simulink subsystem "stack_model_subsystem"  (R2023a)
settings: Solver=VariableStepAuto  StartTime=0.0  StopTime=10.0  RelTol=1e-3
undefined symbols (not defined in the file): constants, coolant_initial_temperature, dewpoint_temperature_degC, env_p, h2_molar_concentration, hydrogen, inlet_flow_lpmin, inlet_pressure_barg, inlet_temperature_degC, oxygen, stack, stack_num_cells, stoichiometry
libraries: fl_lib x28, nesl_utility x26
(part 1 of 2)
settings Model: Creator=stefan.notter  LastModifiedBy=adrian.taveras
settings OptimizationCC: ReuseModelBlockBuffer=off

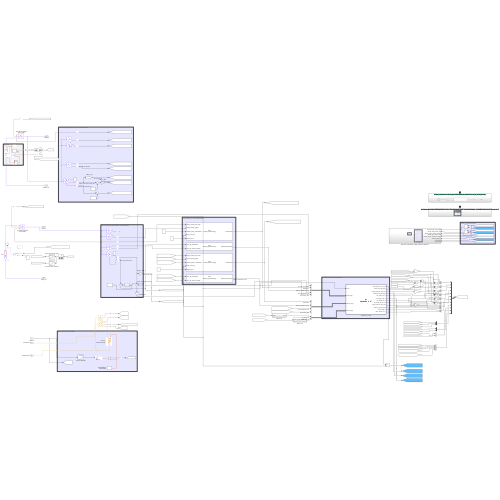
[thumbnail: Simulink's stored preview of the top-level diagram]
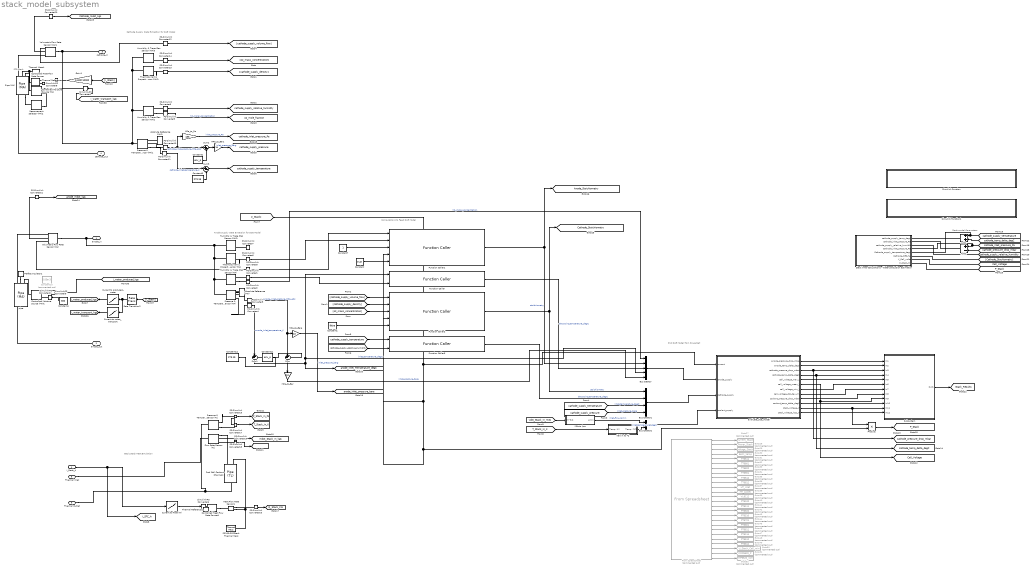
== system stack_model_subsystem ==
  note: Basic Stack Heat Emulation
  note: Computations to Feed DoE Model
  note: Anode Supply Data Extraction for DoE Model
  note: P10 DoE Model from PowerCell
  note: Cathode Supply Data Extraction for DoE Model
  note: FCS-Stack
  note: Stack-model-Parameters
  I_Stack_A : Inport
  Absolute Reference (MA) : fl_lib/Moist Air/Elements/Absolute Reference (MA)
  Absolute Reference (MA)1 : fl_lib/Moist Air/Elements/Absolute Reference (MA)
  Add1 : Sum
  Add2 : Sum  Inputs=+-
  Bus Creator : BusCreator  Inputs=h2_molar_concentration,stoichiometry,dewpoint_temperature_degC,inlet_temperature_degC,inlet_pressure_barg  OutDataTypeStr=Bus: anode_supply
  Bus Creator1 : BusCreator  Inputs=stoichiometry,dewpoint_temperature_degC,inlet_temperature_degC,inlet_pressure_barg  OutDataTypeStr=Bus: cathode_supply
  Bus Creator2 : BusCreator  Inputs=inlet_flow_lpmin,inlet_temperature_degC  OutDataTypeStr=Bus: coolant_supply
  Constant : Constant  Value=true  OutDataTypeStr=boolean
  Constant1 : Constant  Value=false  OutDataTypeStr=boolean
  Constant10 : Constant  Commented=on  Value=0.05e-3
  Constant11 : Constant  Value=env_p
  Constant12 : Constant  Value=273.15
  Constant2 : Constant  Value=env_p
  Constant3 : Constant  Value=273.15
  Constant4 : Constant  Value=300
  Constant7 : Constant
  Controlled Heat Flow Rate Source : fl_lib/Thermal/Thermal Sources/Controlled Heat Flow Rate Source
  Controlled Heat Flow Rate Source1 : fl_lib/Thermal/Thermal Sources/Controlled Heat Flow Rate Source
  Controlled Moisture Source (MA) : fl_lib/Moist Air/Sources/Moisture & Trace Gas Sources/Controlled Moisture Source (MA)  moisture_source_spec=foundation.enum.moisture_source_spec.vapor  Phi_S_specify=off  Phi_S_priority=None  Phi_S=0 kW  Phi_S_nominal_specify=off  Phi_S_nominal_unit=kW  Phi_S_nominal_value=1  mdot_w_S_specify=off  mdot_w_S_priority=None  mdot_w_S=0 kg/s  mdot_w_S_nominal_specify=off  mdot_w_S_nominal_unit=kg/s  mdot_w_S_nominal_value=1
      settings: InternalSimscapePortConfiguration="{\"Bottom\":[],\"Left\":[{\"id\":\"S\",\"label\":\"S\",\"type\":\"foundation.moist_air.moist_air_source\"}],\"Right\":[{\"id\":\"M\",\"label\":\"M\",\"type\":\"input\"},{\"id\":\"T\",\"label\":\"T\",\"type\":\"input\"}],\"Top\":[]}"
  Controlled Moisture Source (MA)1 : fl_lib/Moist Air/Sources/Moisture & Trace Gas Sources/Controlled Moisture Source (MA)  moisture_source_spec=foundation.enum.moisture_source_spec.vapor  Phi_S_specify=off  Phi_S_priority=None  Phi_S=0 kW  Phi_S_nominal_specify=off  Phi_S_nominal_unit=kW  Phi_S_nominal_value=1  mdot_w_S_specify=off  mdot_w_S_priority=None  mdot_w_S=0 kg/s  mdot_w_S_nominal_specify=off  mdot_w_S_nominal_unit=kg/s  mdot_w_S_nominal_value=1
      settings: InternalSimscapePortConfiguration="{\"Bottom\":[],\"Left\":[{\"id\":\"S\",\"label\":\"S\",\"type\":\"foundation.moist_air.moist_air_source\"}],\"Right\":[{\"id\":\"M\",\"label\":\"M\",\"type\":\"input\"},{\"id\":\"T\",\"label\":\"T\",\"type\":\"input\"}],\"Top\":[]}"
  Current to Heat (W) : Lookup_n-D  NumberOfTableDimensions=1  BreakpointsForDimension1=[0:50:400]  Table=[0, 9932, 21438, 33442,47123, 59491, 77033, 93585, 112042]  InternalRulePriority=Speed  RndMeth=Simplest
  Current to produced_water : Lookup_n-D  NumberOfTableDimensions=1  BreakpointsForDimension1=[0;100;200;400;600]  Table=[0;6.491e-6;1.132e-5;1.762e-5;2.762e-5]  InternalRulePriority=Speed  RndMeth=Simplest
  Current to water_transport : Lookup_n-D  NumberOfTableDimensions=1  BreakpointsForDimension1=[0;100;200;400;600]  Table=[0;4.247e-3;8.494e-3;1.697e-2;2.548e-2]  InternalRulePriority=Speed  RndMeth=Simplest
  Flow Rate Sensor (TL) : fl_lib/Thermal Liquid/Sensors/Flow Rate Sensor (TL)  mass_flow_measure=true  volumetric_flow_measure=true  energy_flow_measure=false
      settings: InternalSimscapePortConfiguration="{\"Bottom\":[],\"Left\":[{\"id\":\"A\",\"label\":\"A\",\"type\":\"foundation.thermal_liquid.thermal_liquid\"}],\"Right\":[{\"id\":\"B\",\"label\":\"B\",\"type\":\"foundation.thermal_liquid.thermal_liquid\"},{\"id\":\"M\",\"label\":\"M\",\"type\":\"output\"},{\"id\":\"V\",\"label\":\"V\",\"type\":\"output\"}],\"Top\":[]}"
  From Spreadsheet : FromSpreadsheet  Commented=on  FileName=20231018_14_31_59_ATP.xlsx  Range=A1:AA473537  ExtrapolationAfterLastDataPoint=Hold last value
  Fuel Cell Coolant Channels : fl_lib/Thermal Liquid/Elements/Pipe (TL)  length=sqrt(stack.area) * stack.coolant_num_passes cm  area=stack.coolant_w_channels^2 * stack.coolant_num_layers cm^2  Dh=stack.coolant_w_channels cm  length_add=10 cm  roughness=15e-5 m  Re_lam=2000  Re_tur=4000  shape_factor=64  Nu_lam=3.66  dynamic_compressibility=simscape.enum.onoff.on  inertia=simscape.enum.onoff.off  p0=coolant_initial_pressure MPa  T0=coolant_initial_temperature K  mdot0=0 kg/s
  Function Caller : FunctionCaller  FunctionPrototype=dewpoint_temperature = dewpoint_approximation(moist_air_temperature,moist_air_relative_humidity)  InputArgumentSpecifications=<Enter example>  OutputArgumentSpecifications=<Enter example>
  Function Caller1 : FunctionCaller  FunctionPrototype=stoichiometry = compute_stoichiometry(supply_volume_flow_m3ps,supply_density_kgpm3,reactant_mass_concentration,stack_current_A,isanode_bool)  InputArgumentSpecifications=<Enter example>  OutputArgumentSpecifications=<Enter example>
  Function Caller2 : FunctionCaller  FunctionPrototype=stoichiometry = compute_stoichiometry(supply_volume_flow_m3ps,supply_density_kgpm3,reactant_mass_concentration,stack_current_A,isanode_bool)  InputArgumentSpecifications=<Enter example>  OutputArgumentSpecifications=<Enter example>
  Function Caller3 : FunctionCaller  FunctionPrototype=dewpoint_temperature = dewpoint_approximation(moist_air_temperature,moist_air_relative_humidity)  InputArgumentSpecifications=<Enter example>  OutputArgumentSpecifications=<Enter example>
  Gain1 : Gain  Gain=1/400*10000
  Goto27 : Goto  Commented=on  GotoTag=Current_Stack  TagVisibility=global
  Goto28 : Goto  Commented=on  GotoTag=Power_Stack  TagVisibility=global
  Goto29 : Goto  Commented=on  GotoTag=voltage_Stack  TagVisibility=global
  Goto30 : Goto  Commented=on  GotoTag=EACi_temp  TagVisibility=global
  Goto31 : Goto  Commented=on  GotoTag=TT6511  TagVisibility=global
  Goto32 : Goto  Commented=on  GotoTag=TT6801  TagVisibility=global
  Goto33 : Goto  Commented=on  GotoTag=TT6820  TagVisibility=global
  Goto34 : Goto  Commented=on  GotoTag=TT6901  TagVisibility=global
  Goto35 : Goto  Commented=on  GotoTag=TT6512  TagVisibility=global
  Goto36 : Goto  Commented=on  GotoTag=TT6812  TagVisibility=global
  Goto37 : Goto  Commented=on  GotoTag=HT_inlet  TagVisibility=global
  Goto38 : Goto  Commented=on  GotoTag=HT_outlet  TagVisibility=global
  Goto39 : Goto  Commented=on  GotoTag=VL6112  TagVisibility=global
  Goto40 : Goto  Commented=on  GotoTag=PT6100  TagVisibility=global
  Goto41 : Goto  Commented=on  GotoTag=PT6111  TagVisibility=global
  Goto42 : Goto  Commented=on  GotoTag=PT6500  TagVisibility=global
  Goto43 : Goto  Commented=on  GotoTag=PT6510  TagVisibility=global
  Goto44 : Goto  Commented=on  GotoTag=PT6701  TagVisibility=global
  Goto45 : Goto  Commented=on  GotoTag=PT6801  TagVisibility=global
  Goto46 : Goto  Commented=on  GotoTag=PT6811  TagVisibility=global
  Goto47 : Goto  Commented=on  GotoTag=PT6114  TagVisibility=global
  Goto48 : Goto  Commented=on  GotoTag=PT6512  TagVisibility=global
  Goto49 : Goto  Commented=on  GotoTag=PT6812  TagVisibility=global
  Goto50 : Goto  Commented=on  GotoTag=U_Stack_Cell_min  TagVisibility=global
  Goto51 : Goto  Commented=on  GotoTag=CMP6520_P  TagVisibility=global
  Goto52 : Goto  Commented=on  GotoTag=CMP6520_rpm  TagVisibility=global
  Heat Flow Rate Sensor1 : fl_lib/Thermal/Thermal Sensors/Heat Flow Rate Sensor
  Humidity & Trace Gas Sensor (MA) : fl_lib/Moist Air/Sensors/Humidity & Trace Gas Sensor (MA)  moisture_on=true  moisture_spec=foundation.enum.moisture_spec.relative_humidity  trace_gas_on=true  trace_gas_spec=foundation.enum.trace_gas_spec.mole_fraction
      settings: InternalSimscapePortConfiguration="{\"Bottom\":[],\"Left\":[{\"id\":\"A\",\"label\":\"A\",\"type\":\"foundation.moist_air.moist_air\"}],\"Right\":[{\"id\":\"W\",\"label\":\"W\",\"type\":\"output\"},{\"id\":\"G\",\"label\":\"G\",\"type\":\"output\"}],\"Top\":[]}"
  Humidity & Trace Gas Sensor (MA)1 : fl_lib/Moist Air/Sensors/Humidity & Trace Gas Sensor (MA)  moisture_on=true  moisture_spec=foundation.enum.moisture_spec.relative_humidity  trace_gas_on=true  trace_gas_spec=foundation.enum.trace_gas_spec.mass_fraction
      settings: InternalSimscapePortConfiguration="{\"Bottom\":[],\"Left\":[{\"id\":\"A\",\"label\":\"A\",\"type\":\"foundation.moist_air.moist_air\"}],\"Right\":[{\"id\":\"W\",\"label\":\"W\",\"type\":\"output\"},{\"id\":\"G\",\"label\":\"G\",\"type\":\"output\"}],\"Top\":[]}"
  Humidity & Trace Gas Sensor (MA)2 : fl_lib/Moist Air/Sensors/Humidity & Trace Gas Sensor (MA)  moisture_on=true  moisture_spec=foundation.enum.moisture_spec.relative_humidity  trace_gas_on=true  trace_gas_spec=foundation.enum.trace_gas_spec.mole_fraction
      settings: InternalSimscapePortConfiguration="{\"Bottom\":[],\"Left\":[{\"id\":\"A\",\"label\":\"A\",\"type\":\"foundation.moist_air.moist_air\"}],\"Right\":[{\"id\":\"W\",\"label\":\"W\",\"type\":\"output\"},{\"id\":\"G\",\"label\":\"G\",\"type\":\"output\"}],\"Top\":[]}"
  Humidity & Trace Gas Sensor (MA)3 : fl_lib/Moist Air/Sensors/Humidity & Trace Gas Sensor (MA)  moisture_on=true  moisture_spec=foundation.enum.moisture_spec.relative_humidity  trace_gas_on=true  trace_gas_spec=foundation.enum.trace_gas_spec.mass_fraction
      settings: InternalSimscapePortConfiguration="{\"Bottom\":[],\"Left\":[{\"id\":\"A\",\"label\":\"A\",\"type\":\"foundation.moist_air.moist_air\"}],\"Right\":[{\"id\":\"W\",\"label\":\"W\",\"type\":\"output\"},{\"id\":\"G\",\"label\":\"G\",\"type\":\"output\"}],\"Top\":[]}"
  Kelvin to °C : Subsystem
  M3s to lpm : Subsystem
  MPa_to_Bar : Gain  Gain=10
  MPa_to_Bar1 : Gain  Gain=10
  MPa_to_Bara : Gain  Gain=10
  MPa_to_Pa : Gain  Gain=1e6
  Measurement Selector (MA)2 : fl_lib/Moist Air/Sensors/Measurement Selector (MA)  moisture_spec=foundation.enum.moisture_spec.relative_humidity  trace_gas_spec=foundation.enum.trace_gas_spec.mole_fraction
  PS-Simulink Converter{1..2,4..9,11..14,20..21} (14 alike) : nesl_utility/PS-Simulink Converter  PhysicalDomain=network_engine_domain  SubClassName=ps_output  LeftPortType=input  RightPortType=output  PseudoPeriodic=off  Frequencies=[]  VectorFormat=inherit  Unit=inherit  AffineConversion=off
  PS-Simulink Converter10 : nesl_utility/PS-Simulink Converter  PhysicalDomain=network_engine_domain  SubClassName=ps_output  LeftPortType=input  RightPortType=output  PseudoPeriodic=off  Frequencies=[]  VectorFormat=inherit  Unit=MPa  AffineConversion=off
  PS-Simulink Converter{15,17..19} (4 alike) : nesl_utility/PS-Simulink Converter  PhysicalDomain=network_engine_domain  SubClassName=ps_output  LeftPortType=input  RightPortType=output  PseudoPeriodic=off  Frequencies=[]  VectorFormat=1-D array  Unit=inherit  AffineConversion=off
  PS-Simulink Converter16 : nesl_utility/PS-Simulink Converter  PhysicalDomain=network_engine_domain  SubClassName=ps_output  LeftPortType=input  RightPortType=output  PseudoPeriodic=off  Frequencies=[]  VectorFormat=1-D array  Unit=kW  AffineConversion=off
  PS-Simulink Converter3 : nesl_utility/PS-Simulink Converter  PhysicalDomain=network_engine_domain  SubClassName=ps_output  LeftPortType=input  RightPortType=output  PseudoPeriodic=off  Frequencies=[]  VectorFormat=inherit  Unit=MPa  AffineConversion=off
  PS100-P02Stack Thermal Mass : fl_lib/Thermal/Thermal Elements/Thermal Mass  mass_type=foundation.enum.constant_variable.constant  mass=stack.thermal_mass kg  sp_heat=stack.specific_heat J/kg/K  mass_min=1e-6 kg  num_ports=foundation.enum.numPorts2.one  m_specify=off  m_priority=High  m=1 kg  m_nominal_specify=off  m_nominal_unit=kg  m_nominal_value=1  T_specify=on  T_priority=High  T=coolant_initial_temperature K  T_nominal_specify=off  T_nominal_unit=K  T_nominal_value=1  Q_specify=off  Q_priority=None  Q=20e3 W  Q_nominal_specify=off  Q_nominal_unit=W  Q_nominal_value=1
  Perfect Insulator1 : fl_lib/Thermal/Thermal Elements/Perfect Insulator  T_specify=off  T_priority=None  T=293.15 K  T_nominal_specify=off  T_nominal_unit=K  T_nominal_value=1
  Pipe (MA) : fl_lib/Moist Air/Elements/Pipe (MA)  length=1 m  area=1 m^2  Dh=.1 m  length_add=.1 m  roughness=15e-6 m  Re_lam=2000  Re_tur=4000  shape_factor=1  Nu_lam=3.66  wall_condensation=simscape.enum.onoff.on  RH_ws=1  time_constant=1e-3 s  moisture_trace_gas_source=foundation.enum.moisture_trace_gas_source.controlled  moisture_source_spec=foundation.enum.moisture_source_spec.vapor  moisture_mass_flow=0 kg/s  moisture_temperature_spec=foundation.enum.temperature_spec.atmospheric  moisture_temperature=293.15 K  trace_gas_mass_flow=0 kg/s  trace_gas_temperature_spec=foundation.enum.temperature_spec.atmospheric  trace_gas_temperature=293.15 K  p_I_specify=off  p_I_priority=High  p_I=0.101325 MPa  p_I_nominal_specify=off  p_I_nominal_unit=MPa  p_I_nominal_value=1  T_I_specify=off  T_I_priority=High  T_I=293.15 K  T_I_nominal_specify=off  T_I_nominal_unit=K  T_I_nominal_value=1  RH_I_specify=off  RH_I_priority=High  RH_I=0  RH_I_nominal_specify=off  RH_I_nominal_unit=1  RH_I_nominal_value=1  x_w_I_specify=off  x_w_I_priority=None  x_w_I=0  x_w_I_nominal_specify=off  x_w_I_nominal_unit=1  x_w_I_nominal_value=1  y_w_I_specify=off  y_w_I_priority=None  y_w_I=0  y_w_I_nominal_specify=off  y_w_I_nominal_unit=1  y_w_I_nominal_value=1  HR_I_specify=off  HR_I_priority=None  HR_I=0  HR_I_nominal_specify=off  HR_I_nominal_unit=1  HR_I_nominal_value=1  x_g_I_specify=off  x_g_I_priority=High  x_g_I=0  x_g_I_nominal_specify=off  x_g_I_nominal_unit=1  x_g_I_nominal_value=1  y_g_I_specify=off  y_g_I_priority=None  y_g_I=0  y_g_I_nominal_specify=off  y_g_I_nominal_unit=1  y_g_I_nominal_value=1
      settings: InternalSimscapePortConfiguration="{\"Bottom\":[],\"Left\":[{\"id\":\"A\",\"label\":\"A\",\"type\":\"foundation.moist_air.moist_air\"},{\"id\":\"H\",\"label\":\"H\",\"type\":\"foundation.thermal.thermal\"},{\"id\":\"S\",\"label\":\"S\",\"type\":\"foundation.moist_air.moist_air_source\"}],\"Right\":[{\"id\":\"B\",\"label\":\"B\",\"type\":\"foundation.moist_air.moist_air\"},{\"id\":\"W\",\"label\":\"W\",\"type\":\"output\"},{\"id\":\"F\",\"label\":\"F\",\"type\":\"output\"}],\"Top\":[]}"
  Pressure & Temperature Sensor (MA) : fl_lib/Moist Air/Sensors/Pressure & Temperature Sensor (MA)  reference=foundation.enum.MeasurementReference.difference  pressure=true  pressure_spec=foundation.enum.PressureMeasementSpec.Absolute  temperature=true
      settings: InternalSimscapePortConfiguration="{\"Bottom\":[{\"id\":\"T\",\"label\":\"T\",\"type\":\"output\"}],\"Left\":[{\"id\":\"A\",\"label\":\"A\",\"type\":\"foundation.moist_air.moist_air\"}],\"Right\":[{\"id\":\"B\",\"label\":\"B\",\"type\":\"foundation.moist_air.moist_air\"},{\"id\":\"P\",\"label\":\"P\",\"type\":\"output\"}],\"Top\":[]}"
  Pressure & Temperature Sensor (MA)1 : fl_lib/Moist Air/Sensors/Pressure & Temperature Sensor (MA)  reference=foundation.enum.MeasurementReference.difference  pressure=true  pressure_spec=foundation.enum.PressureMeasementSpec.Absolute  temperature=true
      settings: InternalSimscapePortConfiguration="{\"Bottom\":[{\"id\":\"T\",\"label\":\"T\",\"type\":\"output\"}],\"Left\":[{\"id\":\"A\",\"label\":\"A\",\"type\":\"foundation.moist_air.moist_air\"}],\"Right\":[{\"id\":\"B\",\"label\":\"B\",\"type\":\"foundation.moist_air.moist_air\"},{\"id\":\"P\",\"label\":\"P\",\"type\":\"output\"}],\"Top\":[]}"
  Pressure & Temperature Sensor (TL) : fl_lib/Thermal Liquid/Sensors/Pressure & Temperature Sensor (TL)  reference=foundation.enum.MeasurementReference.absolute  pressure=true  pressure_spec=foundation.enum.PressureMeasementSpec.Absolute  temperature=true
      settings: InternalSimscapePortConfiguration="{\"Bottom\":[{\"id\":\"T\",\"label\":\"T\",\"type\":\"output\"}],\"Left\":[{\"id\":\"A\",\"label\":\"A\",\"type\":\"foundation.thermal_liquid.thermal_liquid\"}],\"Right\":[{\"id\":\"Pa\",\"label\":\"Pa\",\"type\":\"output\"}],\"Top\":[]}"
  Product : Product
  Rate Transition2 : RateTransition
  Simulink Function : Subsystem  TreatAsAtomicUnit=on
  Simulink Function1 : Subsystem  TreatAsAtomicUnit=on
  Simulink-PS Converter1 : nesl_utility/Simulink-PS Converter  PhysicalDomain=network_engine_domain  SubClassName=ps_input  LeftPortType=input  RightPortType=output  PseudoPeriodic=off  Frequencies=[]  NoiseDistribution=none  NoiseParameters=[]  Unit=1  AffineConversion=off  FilteringAndDerivatives=provide  SimscapeFilterOrder=1  InputFilterTimeConstant=0.001  UdotUserProvided=0
  Simulink-PS Converter11 : nesl_utility/Simulink-PS Converter  PhysicalDomain=network_engine_domain  SubClassName=ps_input  LeftPortType=input  RightPortType=output  PseudoPeriodic=off  Frequencies=[]  NoiseDistribution=none  NoiseParameters=[]  Unit=1  AffineConversion=off  FilteringAndDerivatives=provide  SimscapeFilterOrder=1  InputFilterTimeConstant=0.001  UdotUserProvided=0
  Simulink-PS Converter6 : nesl_utility/Simulink-PS Converter  PhysicalDomain=network_engine_domain  SubClassName=ps_input  LeftPortType=input  RightPortType=output  PseudoPeriodic=off  Frequencies=[]  NoiseDistribution=none  NoiseParameters=[]  Unit=J/s  AffineConversion=off  FilteringAndDerivatives=provide  SimscapeFilterOrder=1  InputFilterTimeConstant=0.001  UdotUserProvided=0
  Simulink-PS Converter8 : nesl_utility/Simulink-PS Converter  PhysicalDomain=network_engine_domain  SubClassName=ps_input  LeftPortType=input  RightPortType=output  PseudoPeriodic=off  Frequencies=[]  NoiseDistribution=none  NoiseParameters=[]  Unit=W  AffineConversion=off  FilteringAndDerivatives=provide  SimscapeFilterOrder=1  InputFilterTimeConstant=0.001  UdotUserProvided=0
  Simulink-PS Converter9 : nesl_utility/Simulink-PS Converter  PhysicalDomain=network_engine_domain  SubClassName=ps_input  LeftPortType=input  RightPortType=output  PseudoPeriodic=off  Frequencies=[]  NoiseDistribution=none  NoiseParameters=[]  Unit=1  AffineConversion=off  FilteringAndDerivatives=zero  SimscapeFilterOrder=1  InputFilterTimeConstant=0.001  UdotUserProvided=0
  Stack Inner Calculations - Water production estimation : Subsystem
  Subsystem : Subsystem
  Sum{,1..3} (4 alike) : Sum  Inputs=|+-
  Thermal Mass4 : fl_lib/Thermal/Thermal Elements/Thermal Mass  mass_type=foundation.enum.constant_variable.constant  mass=10 kg  sp_heat=447 J/(K*kg)  mass_min=1e-6 kg  num_ports=foundation.enum.numPorts2.one  m_specify=off  m_priority=High  m=1 kg  m_nominal_specify=off  m_nominal_unit=kg  m_nominal_value=1  T_specify=off  T_priority=High  T=300 K  T_nominal_specify=off  T_nominal_unit=K  T_nominal_value=1  Q_specify=off  Q_priority=None  Q=0 W  Q_nominal_specify=off  Q_nominal_unit=W  Q_nominal_value=1
  Thermal Reference : fl_lib/Thermal/Thermal Elements/Thermal Reference
  Thermal Reference1 : fl_lib/Thermal/Thermal Elements/Thermal Reference
  Thermodynamic Properties Sensor (MA) : fl_lib/Moist Air/Sensors/Thermodynamic Properties Sensor (MA)  measurement_mass_spec=foundation.enum.measurement_mass_spec.mixture  enthalpy=true  density=true  specific_heat=true  entropy=true
      settings: InternalSimscapePortConfiguration="{\"Bottom\":[{\"id\":\"CP\",\"label\":\"cp\",\"type\":\"output\"},{\"id\":\"S\",\"label\":\"s\",\"type\":\"output\"}],\"Left\":[{\"id\":\"A\",\"label\":\"A\",\"type\":\"foundation.moist_air.moist_air\"}],\"Right\":[{\"id\":\"H\",\"label\":\"h\",\"type\":\"output\"},{\"id\":\"RHO\",\"label\":\"ρ\",\"type\":\"output\"}],\"Top\":[]}"
  Thermodynamic Properties Sensor (MA)1 : fl_lib/Moist Air/Sensors/Thermodynamic Properties Sensor (MA)  measurement_mass_spec=foundation.enum.measurement_mass_spec.mixture  enthalpy=true  density=true  specific_heat=true  entropy=true
      settings: InternalSimscapePortConfiguration="{\"Bottom\":[{\"id\":\"CP\",\"label\":\"cp\",\"type\":\"output\"},{\"id\":\"S\",\"label\":\"s\",\"type\":\"output\"}],\"Left\":[{\"id\":\"A\",\"label\":\"A\",\"type\":\"foundation.moist_air.moist_air\"}],\"Right\":[{\"id\":\"H\",\"label\":\"h\",\"type\":\"output\"},{\"id\":\"RHO\",\"label\":\"ρ\",\"type\":\"output\"}],\"Top\":[]}"
  Volumetric Flow Rate Sensor (MA) : fl_lib/Moist Air/Sensors/Flow Rate Sensor (MA)  mass_flow_measure=true  volumetric_flow_measure=true  volumetric_flow_conditions=foundation.enum.volumetric_flow_conditions.actual  p_std=0.101325 MPa  T_std=20 degC  RH_std=0.65  energy_flow_measure=false  vapor_flow_measure=false  gas_flow_measure=false
      settings: InternalSimscapePortConfiguration="{\"Bottom\":[],\"Left\":[{\"id\":\"A\",\"label\":\"A\",\"type\":\"foundation.moist_air.moist_air\"}],\"Right\":[{\"id\":\"B\",\"label\":\"B\",\"type\":\"foundation.moist_air.moist_air\"},{\"id\":\"M\",\"label\":\"M\",\"type\":\"output\"},{\"id\":\"V\",\"label\":\"V\",\"type\":\"output\"}],\"Top\":[]}"
  Volumetric Flow Rate Sensor (MA)1 : fl_lib/Moist Air/Sensors/Flow Rate Sensor (MA)  mass_flow_measure=true  volumetric_flow_measure=true  volumetric_flow_conditions=foundation.enum.volumetric_flow_conditions.actual  p_std=0.101325 MPa  T_std=20 degC  RH_std=0.65  energy_flow_measure=false  vapor_flow_measure=false  gas_flow_measure=false
      settings: InternalSimscapePortConfiguration="{\"Bottom\":[],\"Left\":[{\"id\":\"A\",\"label\":\"A\",\"type\":\"foundation.moist_air.moist_air\"}],\"Right\":[{\"id\":\"B\",\"label\":\"B\",\"type\":\"foundation.moist_air.moist_air\"},{\"id\":\"M\",\"label\":\"M\",\"type\":\"output\"},{\"id\":\"V\",\"label\":\"V\",\"type\":\"output\"}],\"Top\":[]}"
  evaluate_doe_model : MATLAB Function  TreatAsAtomicUnit=on  SystemSampleTime=1
  pipe : fl_lib/Moist Air/Elements/Pipe (MA)  length=0.25 m  area=pi*0.05^2/4 m^2  Dh=0.05 m  length_add=0.1 m  roughness=15e-6 m  Re_lam=2000  Re_tur=4000  shape_factor=64  Nu_lam=3.66  wall_condensation=simscape.enum.onoff.off  RH_ws=1  time_constant=1e-3 s  moisture_trace_gas_source=foundation.enum.moisture_trace_gas_source.controlled  moisture_source_spec=foundation.enum.moisture_source_spec.vapor  moisture_mass_flow=0 kg/s  moisture_temperature_spec=foundation.enum.temperature_spec.atmospheric  moisture_temperature=293.15 K  trace_gas_mass_flow=0 kg/s  trace_gas_temperature_spec=foundation.enum.temperature_spec.atmospheric  trace_gas_temperature=293.15 K  p_I_specify=off  p_I_priority=High  p_I=env_p MPa  p_I_nominal_specify=off  p_I_nominal_unit=MPa  p_I_nominal_value=1  T_I_specify=off  T_I_priority=High  T_I=env_T degC  T_I_nominal_specify=off  T_I_nominal_unit=K  T_I_nominal_value=1  RH_I_specify=on  RH_I_priority=High  RH_I=0.0005  RH_I_nominal_specify=off  RH_I_nominal_unit=1  RH_I_nominal_value=1  x_w_I_specify=off  x_w_I_priority=None  x_w_I=0  x_w_I_nominal_specify=off  x_w_I_nominal_unit=1  x_w_I_nominal_value=1  y_w_I_specify=off  y_w_I_priority=None  y_w_I=0  y_w_I_nominal_specify=off  y_w_I_nominal_unit=1  y_w_I_nominal_value=1  HR_I_specify=off  HR_I_priority=None  HR_I=0  HR_I_nominal_specify=off  HR_I_nominal_unit=1  HR_I_nominal_value=1  x_g_I_specify=off  x_g_I_priority=None  x_g_I=0  x_g_I_nominal_specify=off  x_g_I_nominal_unit=1  x_g_I_nominal_value=1  y_g_I_specify=off  y_g_I_priority=High  y_g_I=tank_yH2  y_g_I_nominal_specify=off  y_g_I_nominal_unit=1  y_g_I_nominal_value=1
      settings: InternalSimscapePortConfiguration="{\"Bottom\":[],\"Left\":[{\"id\":\"A\",\"label\":\"A\",\"type\":\"foundation.moist_air.moist_air\"},{\"id\":\"H\",\"label\":\"H\",\"type\":\"foundation.thermal.thermal\"},{\"id\":\"S\",\"label\":\"S\",\"type\":\"foundation.moist_air.moist_air_source\"}],\"Right\":[{\"id\":\"B\",\"label\":\"B\",\"type\":\"foundation.moist_air.moist_air\"},{\"id\":\"W\",\"label\":\"W\",\"type\":\"output\"},{\"id\":\"F\",\"label\":\"F\",\"type\":\"output\"}],\"Top\":[]}"
  anode_in : PMIOPort  Side=Left
  anode_out : PMIOPort  Port=2  Side=Left
  cathode_in : PMIOPort  Port=3  Side=Right
  cathode_out : PMIOPort  Port=4  Side=Right
  Thermal Inlet : PMIOPort  Port=5  Side=Left
  Thermal Outlet : PMIOPort  Port=6  Side=Left
  tag scope: Anode_Stoichiometry=global, Cathode_Stoichiometry=global, Cathode_mdot_kgs=global, Cell_Voltage=global, I_SFC_A=global, P_Stack=global, P_Stack_in_Pa=global, Q_Stack_kW=global, Stack_Results=global, T_Stack_in_K=global, anode_inlet_Temperature_degC=global, anode_inlet_pressure_bara=global, anode_mdot_kgs=global, cathode_inlet_pressure_Pa=global, cathode_pressure_drop_mbar=global, cathode_supply_pressure=global, cathode_supply_relative_humidity=global, cathode_supply_temperature=global, cathode_temp_delta_degC=global, i_water_produced_kgs=global, i_water_transport_kgs=global, mdot_Stack_in_kgs=global, o2_mole_fraction=global, vdot_Stack_in_m3s=global
  wires:
  evaluate_doe_model/11(stack_voltage_V) -> Subsystem/11(In11), Product/1
  Bus Creator/1 -> evaluate_doe_model/2(anode_supply)
  Function Caller1/1 -> [Anode_Stoichiometry], Bus Creator/2  "stoichiometry"
  Function Caller/1 -> Bus Creator/3  "dewpoint_temperature_degC"
  [cathode_supply_pressure] -> Bus Creator1/4  "inlet_pressure_barg"
  [cathode_supply_temperature] -> Bus Creator1/3  "inlet_temperature_degC"
  Function Caller3/1 -> Bus Creator1/2  "dewpoint_temperature_degC"
  Function Caller2/1 -> [Cathode_Stoichiometry], Bus Creator1/1  "stoichiometry"
  Bus Creator1/1 -> evaluate_doe_model/3(cathode_supply)
  Bus Creator2/1 -> evaluate_doe_model/4(coolant_supply)
  M3s to lpm/1(L/min) -> Bus Creator2/1  "inlet_flow_lpmin"
  Kelvin to °C/1(Temp. (°C)) -> Bus Creator2/2  "inlet_temperature_degC"
  [i_Stack] -> evaluate_doe_model/1(current), Function Caller1/4, Product/2, Function Caller2/4
  PS-Simulink Converter3/1 -> MPa_to_Bara/1, Sum/1  "anode_inlet_pressure_MPa_abs"
  Constant11/1 -> Sum/2
  Sum/1 -> MPa_to_Bar/1
  PS-Simulink Converter4/1 -> Sum1/1  "anode_inlet_temperature_K"
  Constant12/1 -> Sum1/2
  PS-Simulink Converter2/1 -> Bus Creator/1  "h2_molar_concentration"
  MPa_to_Bar/1 -> Bus Creator/5  "inlet_pressure_barg"
  Sum1/1 -> Bus Creator/4, Function Caller/1, [anode_inlet_Temperature_degC]  "inlet_temperature_degC"
  PS-Simulink Converter1/1 -> Function Caller/2
  PS-Simulink Converter5/1 -> Function Caller1/1
  Constant/1 -> Function Caller1/5
  PS-Simulink Converter6/1 -> Function Caller1/2
  Constant1/1 -> Function Caller2/5
  PS-Simulink Converter10/1 -> Sum2/1, MPa_to_Pa/1  "cathode_inlet_pressure_MPa_abs"
  Constant2/1 -> Sum2/2
  PS-Simulink Converter11/1 -> Sum3/1  "cathode_inlet_temperature_K"
  Constant3/1 -> Sum3/2
  PS-Simulink Converter14/1 -> [o2_mass_concentration]
  PS-Simulink Converter13/1 -> [cathode_supply_density]
  PS-Simulink Converter8/1 -> [cathode_supply_relative_humidity]
  PS-Simulink Converter9/1 -> [o2_mole_fraction]  "h2_molar_concentration"
  PS-Simulink Converter12/1 -> [cathode_supply_volume_flow]
  [o2_mass_concentration] -> Function Caller2/3
  [cathode_supply_density] -> Function Caller2/2
  [cathode_supply_volume_flow] -> Function Caller2/1
  Sum2/1 -> MPa_to_Bar1/1
  MPa_to_Bar1/1 -> [cathode_supply_pressure]  "inlet_pressure_barg"
  Sum3/1 -> [cathode_supply_temperature]
  [cathode_supply_temperature] -> Function Caller3/1
  [cathode_supply_relative_humidity] -> Function Caller3/2
  [T_Stack_in_K] -> Kelvin to °C/1(Temp. (K))
  [vdot_Stack_in_m3s] -> M3s to lpm/1(M^3/S)
  I_Stack_A/1 -> [I_SFC_A], Current to Heat (W)/1
  PS-Simulink Converter16/1 -> [Q_Stack_kW]
  Current to Heat (W)/1 -> Simulink-PS Converter6/1
  PS-Simulink Converter17/1 -> [T_Stack_in_K]
  PS-Simulink Converter18/1 -> [mdot_Stack_in_kgs]
  PS-Simulink Converter19/1 -> [vdot_Stack_in_m3s]
  Constant4/1 -> Simulink-PS Converter11/1
  [i_Stack] -> Gain1/1
  Gain1/1 -> Simulink-PS Converter8/1
  evaluate_doe_model/3(cathode_pressure_drop_mbar) -> Subsystem/3(In3), [cathode_pressure_drop_mbar]
  evaluate_doe_model/6(cell_voltage_mean_V) -> Subsystem/9(In9), [Cell_Voltage]
  [cathode_supply_relative_humidity] -> Stack Inner Calculations - Water production estimation/3(cathode_supply_relative_humidity)
  [Cathode_Stochiometry] -> Stack Inner Calculations - Water production estimation/6(Cathode_OER_%)
  [Cell_Voltage] -> Stack Inner Calculations - Water production estimation/7(V_Cell_volts)
  [cathode_inlet_pressure_Pa] -> Stack Inner Calculations - Water production estimation/4(Cathode_inlet_pressure_Pa), Add2/1
  Add1/1 -> Stack Inner Calculations - Water production estimation/1(cathode_supply_temp_degC)
  [cathode_supply_temperature] -> Stack Inner Calculations - Water production estimation/5(Cathode_supply_temperature_degC), Add1/1
  Add2/1 -> Stack Inner Calculations - Water production estimation/2(cathode_inlet_pressure_Pa)
  [cathode_pressure_drop_mbar] -> Add2/2
  [P_Stack] -> Stack Inner Calculations - Water production estimation/8(P_Stack_W)
  [cathode_temp_delta_degC] -> Add1/2
  MPa_to_Pa/1 -> [cathode_inlet_pressure_Pa]  "inlet_pressure_Pa"
  Product/1 -> [P_Stack]
  MPa_to_Bara/1 -> [anode_inlet_pressure_bara]  "inlet_pressure_barg"
  PS-Simulink Converter15/1 -> [P_Stack_in_Pa]
  PS-Simulink Converter20/1 -> [Cathode_mdot_kgs]
  PS-Simulink Converter21/1 -> [anode_mdot_kgs]
  evaluate_doe_model/4(cathode_temp_delta_degC) -> Subsystem/4(In4), [cathode_temp_delta_degC]
  [i_water_transport_kgs] -> Simulink-PS Converter1/1
  Current to water_transport/1 -> [i_water_transport_kgs]
  Current to produced_water/1 -> [i_water_produced_kgs]
  [i_Stack] -> Rate Transition2/1
  Rate Transition2/1 -> Current to produced_water/1, Current to water_transport/1
  [i_water_produced_kgs] -> Simulink-PS Converter9/1
  Constant7/1 -> Function Caller1/3
  From Spreadsheet/9 -> Goto35/1
  From Spreadsheet/11 -> Goto37/1
  From Spreadsheet/17 -> Goto43/1
  From Spreadsheet/16 -> Goto42/1
  From Spreadsheet/18 -> Goto44/1
  From Spreadsheet/19 -> Goto45/1
  From Spreadsheet/5 -> Goto31/1
  From Spreadsheet/4 -> Goto30/1
  From Spreadsheet/6 -> Goto32/1
  From Spreadsheet/8 -> Goto34/1
  From Spreadsheet/22 -> Goto48/1
  From Spreadsheet/10 -> Goto36/1
  From Spreadsheet/26 -> Goto52/1
  From Spreadsheet/14 -> Goto40/1
  From Spreadsheet/12 -> Goto38/1
  From Spreadsheet/23 -> Goto49/1
  From Spreadsheet/7 -> Goto33/1
  From Spreadsheet/24 -> Goto50/1
  From Spreadsheet/15 -> Goto41/1
  From Spreadsheet/3 -> Goto29/1
  From Spreadsheet/20 -> Goto46/1
  From Spreadsheet/25 -> Goto51/1
  From Spreadsheet/1 -> Goto27/1
  From Spreadsheet/13 -> Goto39/1
  From Spreadsheet/2 -> Goto28/1
  From Spreadsheet/21 -> Goto47/1
  evaluate_doe_model/1(anode_pressure_drop_mbar) -> Subsystem/1(In1)
  evaluate_doe_model/2(anode_temp_delta_degC) -> Subsystem/2(In2)
  evaluate_doe_model/5(cell_voltage_max_V) -> Subsystem/5(In5)
  evaluate_doe_model/7(cell_voltage_min_V) -> Subsystem/6(In6)
  evaluate_doe_model/8(cell_voltage_std_dev_mV) -> Subsystem/7(In7)
  evaluate_doe_model/9(coolant_pressure_drop_mbar) -> Subsystem/8(In8)
  evaluate_doe_model/10(coolant_temp_delta_degC) -> Subsystem/10(In10)
  evaluate_doe_model/12(stack_voltage_loss_V) -> Subsystem/12(In12)
  Subsystem/1(Out1) -> [Stack_Results]
  connections:
  anode_in/RConn1 -- Humidity & Trace Gas Sensor (MA)/LConn1 -- Pressure & Temperature Sensor (MA)/LConn1 -- Thermodynamic Properties Sensor (MA)/LConn1 -- Humidity & Trace Gas Sensor (MA)1/LConn1 -- Volumetric Flow Rate Sensor (MA)/LConn1
  Volumetric Flow Rate Sensor (MA)1/LConn1 -- Thermodynamic Properties Sensor (MA)1/LConn1 -- Humidity & Trace Gas Sensor (MA)3/LConn1 -- Humidity & Trace Gas Sensor (MA)2/LConn1 -- Pressure & Temperature Sensor (MA)1/LConn1 -- cathode_in/RConn1
  Fuel Cell Coolant Channels/RConn1 -- Pressure & Temperature Sensor (TL)/LConn1 -- Thermal Outlet/RConn1
  Heat Flow Rate Sensor1/RConn2 -- Fuel Cell Coolant Channels/LConn2 -- PS100-P02Stack Thermal Mass/LConn1
  Controlled Heat Flow Rate Source/LConn1 -- Thermal Mass4/LConn1 -- Pipe (MA)/LConn2
  Measurement Selector (MA)2/RConn2 -- Controlled Moisture Source (MA)/RConn2
  Humidity & Trace Gas Sensor (MA)/RConn2 -- PS-Simulink Converter2/LConn1
  PS-Simulink Converter3/LConn1 -- Pressure & Temperature Sensor (MA)/RConn2
  PS-Simulink Converter4/LConn1 -- Pressure & Temperature Sensor (MA)/RConn3
  Absolute Reference (MA)/LConn1 -- Pressure & Temperature Sensor (MA)/RConn1
  PS-Simulink Converter1/LConn1 -- Humidity & Trace Gas Sensor (MA)/RConn1
  Volumetric Flow Rate Sensor (MA)/RConn3 -- PS-Simulink Converter5/LConn1
  Thermodynamic Properties Sensor (MA)/RConn2 -- PS-Simulink Converter6/LConn1
  PS-Simulink Converter7/LConn1 -- Humidity & Trace Gas Sensor (MA)1/RConn2
  PS-Simulink Converter14/LConn1 -- Humidity & Trace Gas Sensor (MA)3/RConn2
  PS-Simulink Converter8/LConn1 -- Humidity & Trace Gas Sensor (MA)2/RConn1
  PS-Simulink Converter10/LConn1 -- Pressure & Temperature Sensor (MA)1/RConn2
  Absolute Reference (MA)1/LConn1 -- Pressure & Temperature Sensor (MA)1/RConn1
  Humidity & Trace Gas Sensor (MA)2/RConn2 -- PS-Simulink Converter9/LConn1
  Thermodynamic Properties Sensor (MA)1/RConn2 -- PS-Simulink Converter13/LConn1
  Volumetric Flow Rate Sensor (MA)1/RConn3 -- PS-Simulink Converter12/LConn1
  Pressure & Temperature Sensor (MA)1/RConn3 -- PS-Simulink Converter11/LConn1
  pipe/LConn1 -- Volumetric Flow Rate Sensor (MA)/RConn1
  anode_out/RConn1 -- pipe/RConn1
  Thermal Inlet/RConn1 -- Flow Rate Sensor (TL)/LConn1
  Simulink-PS Converter6/RConn1 -- Controlled Heat Flow Rate Source1/RConn1
  Heat Flow Rate Sensor1/RConn1 -- PS-Simulink Converter16/LConn1
  Controlled Heat Flow Rate Source1/LConn1 -- Heat Flow Rate Sensor1/LConn1
  Thermal Reference1/LConn1 -- Controlled Heat Flow Rate Source1/RConn2
  Flow Rate Sensor (TL)/RConn1 -- Fuel Cell Coolant Channels/LConn1
  PS-Simulink Converter18/LConn1 -- Flow Rate Sensor (TL)/RConn2
  PS-Simulink Converter19/LConn1 -- Flow Rate Sensor (TL)/RConn3
  Simulink-PS Converter11/RConn1 -- Controlled Moisture Source (MA)1/RConn2
  Controlled Moisture Source (MA)1/RConn1 -- Simulink-PS Converter9/RConn1
  Controlled Moisture Source (MA)1/LConn1 -- pipe/LConn3
  Perfect Insulator1/LConn1 -- pipe/LConn2
  Simulink-PS Converter8/RConn1 -- Controlled Heat Flow Rate Source/RConn1
  Controlled Moisture Source (MA)/RConn1 -- Simulink-PS Converter1/RConn1
  cathode_out/RConn1 -- Pipe (MA)/RConn1
  Controlled Moisture Source (MA)/LConn1 -- Pipe (MA)/LConn3
  Thermal Reference/LConn1 -- Controlled Heat Flow Rate Source/RConn2
  Pipe (MA)/RConn3 -- Measurement Selector (MA)2/LConn1
  Volumetric Flow Rate Sensor (MA)1/RConn1 -- Pipe (MA)/LConn1
  Pressure & Temperature Sensor (TL)/RConn2 -- PS-Simulink Converter17/LConn1
  Pressure & Temperature Sensor (TL)/RConn1 -- PS-Simulink Converter15/LConn1
  Volumetric Flow Rate Sensor (MA)1/RConn2 -- PS-Simulink Converter20/LConn1
  PS-Simulink Converter21/LConn1 -- Volumetric Flow Rate Sensor (MA)/RConn2

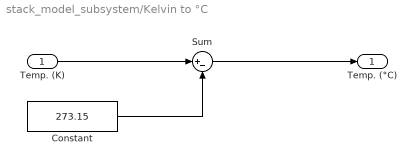
== system stack_model_subsystem/Kelvin to °C ==
  Temp. (K) : Inport
  Constant : Constant  Value=273.15
  Sum : Sum  Inputs=|+-
  Temp. (°C) : Outport
  wires:
  Temp. (K)/1 -> Sum/1
  Sum/1 -> Temp. (°C)/1
  Constant/1 -> Sum/2

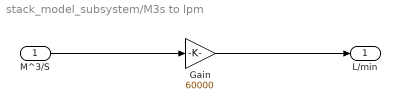
== system stack_model_subsystem/M3s to lpm ==
  M^3/S : Inport
  Gain : Gain  Gain=60000
  L/min : Outport
  wires:
  Gain/1 -> L/min/1
  M^3/S/1 -> Gain/1

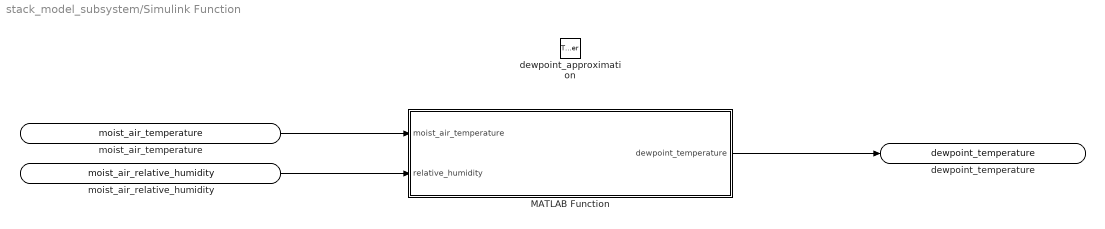
== system stack_model_subsystem/Simulink Function ==
  dewpoint_approximation : TriggerPort  TriggerType=function-call  IsSimulinkFunction=on  FunctionName=dewpoint_approximation  FunctionVisibility=scoped  VariantControl=(inherit)
  MATLAB Function : MATLAB Function  TreatAsAtomicUnit=on
  moist_air_temperature : ArgIn  DisableCoverage=on  ArgumentName=moist_air_temperature
  moist_air_relative_humidity : ArgIn  DisableCoverage=on  Port=2  ArgumentName=moist_air_relative_humidity
  dewpoint_temperature : ArgOut  DisableCoverage=on  ArgumentName=dewpoint_temperature
  wires:
  moist_air_relative_humidity/1 -> MATLAB Function/2(relative_humidity)
  moist_air_temperature/1 -> MATLAB Function/1(moist_air_temperature)
  MATLAB Function/1(dewpoint_temperature) -> dewpoint_temperature/1

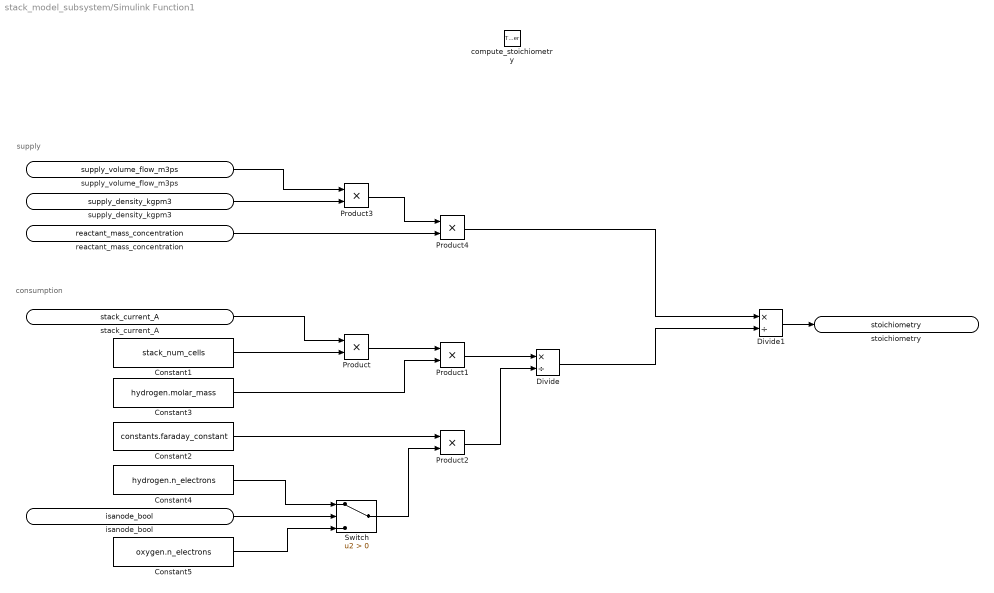
== system stack_model_subsystem/Simulink Function1 ==
  note: consumption
  note: supply
  compute_stoichiometry : TriggerPort  TriggerType=function-call  IsSimulinkFunction=on  FunctionName=compute_stoichiometry  FunctionVisibility=scoped  VariantControl=(inherit)
  Constant1 : Constant  Value=stack_num_cells
  Constant2 : Constant  Value=constants.faraday_constant
  Constant3 : Constant  Value=hydrogen.molar_mass
  Constant4 : Constant  Value=hydrogen.n_electrons
  Constant5 : Constant  Value=oxygen.n_electrons
  Divide : Product  Inputs=*/  RndMeth=Zero  SaturateOnIntegerOverflow=on
  Divide1 : Product  Inputs=*/  RndMeth=Zero  SaturateOnIntegerOverflow=on
  Product{,1..4} (5 alike) : Product
  Switch : Switch  Criteria=u2 > Threshold  SaturateOnIntegerOverflow=off  InputSameDT=off
  supply_volume_flow_m3ps : ArgIn  DisableCoverage=on  ArgumentName=supply_volume_flow_m3ps
  supply_density_kgpm3 : ArgIn  DisableCoverage=on  Port=2  ArgumentName=supply_density_kgpm3
  reactant_mass_concentration : ArgIn  DisableCoverage=on  Port=3  ArgumentName=reactant_mass_concentration
  stack_current_A : ArgIn  DisableCoverage=on  Port=4  ArgumentName=stack_current_A
  isanode_bool : ArgIn  DisableCoverage=on  Port=5  OutDataTypeStr=boolean  ArgumentName=isanode_bool
  stoichiometry : ArgOut  DisableCoverage=on  ArgumentName=stoichiometry
  wires:
  Divide/1 -> Divide1/2
  Product4/1 -> Divide1/1
  Product3/1 -> Product4/1
  reactant_mass_concentration/1 -> Product4/2
  supply_density_kgpm3/1 -> Product3/2
  supply_volume_flow_m3ps/1 -> Product3/1
  Product2/1 -> Divide/2
  Switch/1 -> Product2/2
  Constant5/1 -> Switch/3
  Constant4/1 -> Switch/1
  isanode_bool/1 -> Switch/2
  Constant3/1 -> Product1/2
  Constant2/1 -> Product2/1
  Product1/1 -> Divide/1
  Constant1/1 -> Product/2
  Product/1 -> Product1/1
  Divide1/1 -> stoichiometry/1
  stack_current_A/1 -> Product/1

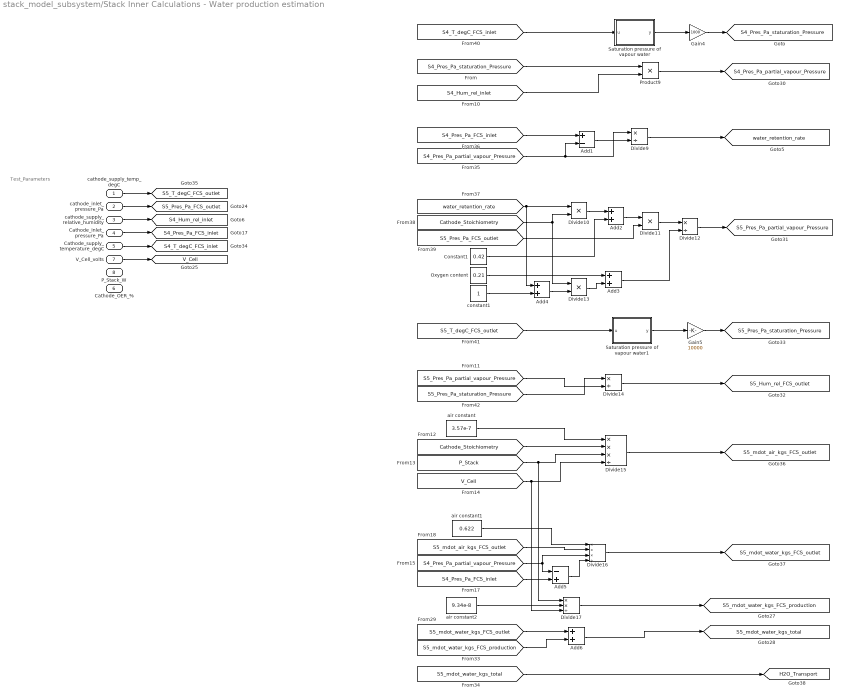
== system stack_model_subsystem/Stack Inner Calculations - Water production estimation ==
  note: Test_Parameters
  cathode_supply_temp_degC : Inport
  cathode_inlet_pressure_Pa : Inport  Port=2
  cathode_supply_relative_humidity : Inport  Port=3
  Cathode_inlet_pressure_Pa : Inport  Port=4
  Cathode_supply_temperature_degC : Inport  Port=5
  Cathode_OER_% : Inport  Port=6
  V_Cell_volts : Inport  Port=7
  P_Stack_W : Inport  Port=8
  Add1 : Sum  Inputs=+-
  Add{2..4,6} (4 alike) : Sum
  Add5 : Sum  Inputs=-+
  Constant1 : Constant  Value=0.42
  Divide10 : Product  Inputs=**
  Divide11 : Product  Inputs=**
  Divide12 : Product  Inputs=*/
  Divide13 : Product  Inputs=**
  Divide14 : Product  Inputs=*/
  Divide15 : Product  Inputs=***/
  Divide16 : Product  Inputs=***/
  Divide17 : Product  Inputs=**/
  Divide9 : Product  Inputs=*/
  Gain4 : Gain  Gain=1000
  Gain5 : Gain  Gain=10000
  Oxygen content : Constant  Value=0.21
  Product9 : Product
  Saturation pressure of vapour water : MATLAB Function  TreatAsAtomicUnit=on
  Saturation pressure of vapour water1 : MATLAB Function  TreatAsAtomicUnit=on
  air constant : Constant  Value=3.57e-7
  air constant1 : Constant  Value=0.622
  air constant2 : Constant  Value=9.34e-8
  constant1 : Constant
  tag scope: H2O_Transport=global, S4_Hum_rel_inlet=global, S4_Pres_Pa_FCS_inlet=global, S4_Pres_Pa_partial_vapour_Pressure=global, S4_Pres_Pa_staturation_Pressure=global, S4_T_degC_FCS_inlet=global, S5_Hum_rel_FCS_outlet=global, S5_Pres_Pa_FCS_outlet=global, S5_Pres_Pa_partial_vapour_Pressure=global, S5_Pres_Pa_staturation_Pressure=global, S5_T_degC_FCS_outlet=global, S5_mdot_air_kgs_FCS_outlet=global, S5_mdot_water_kgs_FCS_outlet=global, S5_mdot_water_kgs_FCS_production=global, S5_mdot_water_kgs_total=global, V_Cell=global, water_retention_rate=global
  wires:
  [S5_Pres_Pa_staturation_Pressure] -> Divide14/1
  [S5_Pres_Pa_partial_vapour_Pressure] -> Divide14/2
  cathode_inlet_pressure_Pa/1 -> [S5_Pres_Pa_FCS_outlet]
  cathode_supply_temp_degC/1 -> [S5_T_degC_FCS_outlet]
  cathode_supply_relative_humidity/1 -> [S4_Hum_rel_inlet]
  [V_Cell] -> Divide15/4, Divide17/3
  Divide10/1 -> Add2/1
  Divide14/1 -> [S5_Hum_rel_FCS_outlet]
  Divide17/1 -> [S5_mdot_water_kgs_FCS_production]
  Divide12/1 -> [S5_Pres_Pa_partial_vapour_Pressure]
  air constant1/1 -> Divide16/1
  Divide16/1 -> [S5_mdot_water_kgs_FCS_outlet]
  [S4_Pres_Pa_FCS_inlet] -> Add1/1
  Cathode_inlet_pressure_Pa/1 -> [S4_Pres_Pa_FCS_inlet]
  Add3/1 -> Divide12/2
  [S4_Pres_Pa_FCS_inlet] -> Add5/2
  V_Cell_volts/1 -> [V_Cell]
  [S4_T_degC_FCS_inlet] -> Saturation pressure of vapour water/1(u)
  Add1/1 -> Divide9/2
  Divide9/1 -> [water_retention_rate]
  Divide15/1 -> [S5_mdot_air_kgs_FCS_outlet]
  Oxygen content/1 -> Add3/1
  Add4/1 -> Divide13/2
  Cathode_supply_temperature_degC/1 -> [S4_T_degC_FCS_inlet]
  Saturation pressure of vapour water/1(y) -> Gain4/1
  Add6/1 -> [S5_mdot_water_kgs_total]
  [S5_Pres_Pa_FCS_outlet] -> Divide11/2
  constant1/1 -> Add4/2
  [S5_mdot_water_kgs_FCS_production] -> Add6/2
  Divide11/1 -> Divide12/1
  Add5/1 -> Divide16/4
  [S4_Pres_Pa_staturation_Pressure] -> Product9/1
  [S4_Hum_rel_inlet] -> Product9/2
  air constant2/1 -> Divide17/2
  [P_Stack] -> Divide15/3, Divide17/1
  [S5_mdot_water_kgs_total] -> [H2O_Transport]
  Divide13/1 -> Add3/2
  [S5_T_degC_FCS_outlet] -> Saturation pressure of vapour water1/1(u)
  [Cathode_Stoichiometry] -> Divide15/2
  [S5_mdot_water_kgs_FCS_outlet] -> Add6/1
  Saturation pressure of vapour water1/1(y) -> Gain5/1
  [S4_Pres_Pa_partial_vapour_Pressure] -> Add1/2, Divide9/1
  Constant1/1 -> Add2/2
  Add2/1 -> Divide11/1
  Gain4/1 -> [S4_Pres_Pa_staturation_Pressure]
  [water_retention_rate] -> Add4/1, Divide10/1
  [Cathode_Stoichiometry] -> Divide10/2, Divide13/1
  [S4_Pres_Pa_partial_vapour_Pressure] -> Add5/1, Divide16/3
  Product9/1 -> [S4_Pres_Pa_partial_vapour_Pressure]
  air constant/1 -> Divide15/1
  Gain5/1 -> [S5_Pres_Pa_staturation_Pressure]
  [S5_mdot_air_kgs_FCS_outlet] -> Divide16/2

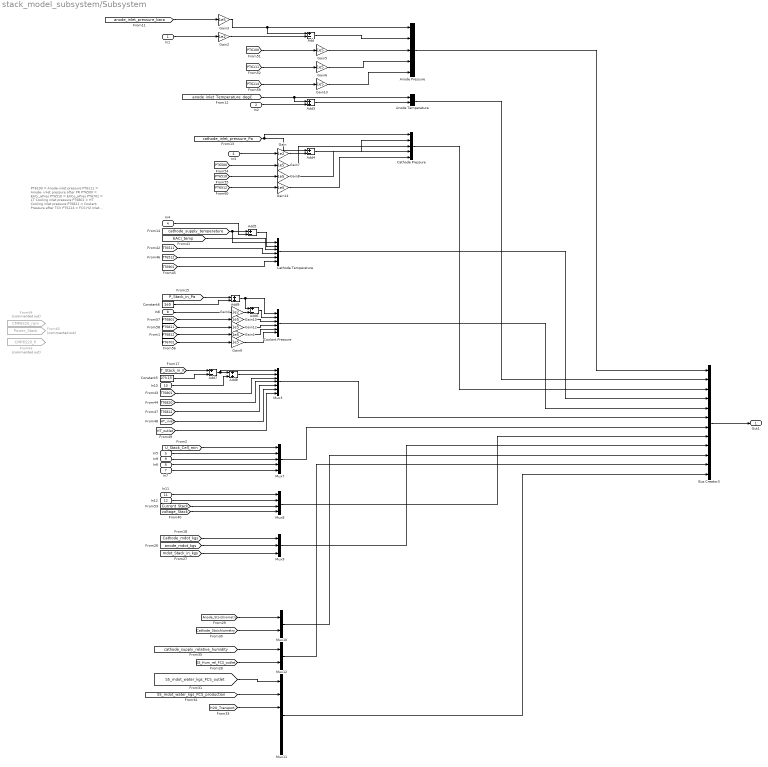
== system stack_model_subsystem/Subsystem ==
  note: PT6100 = Anode-inlet pressure
      | PT6111 = Anode- inlet pressure after PR
      | PT6500 = EACi_aPres
      | PT6510 = EACo_aPres
      | PT6701 = LT Cooling inlet pressure
      | PT6801 = HT Cooling inlet pressure
      | PT6811 = Coolant Pressure after TCV
      | PT6114 = FCS H2 inlet pressure
      | PT6512 = FCS O2 inlet Pressure
      | PT6812 = FCS Coolant inlet pressure
      |
      | TT6100 = Anode- inlet Temperature
      | TT6111 = Anode- after Temperature
      | TT6500 = EACi_Temp
      | TT6510 = EACo_Temp
      | TT6701 = LT Cooling inlet Temperature
      | TT6801 = HT Cooling inlet Temperature
      | TT6811 = Coolant Temperature after TCV
      | TT6114 = FCS H2 inlet Temperature
      | TT6512 = FCS O2 inlet Temperature
      | TT6812 = FCS Coolant inlet Temperature
  In1 : Inport
  In2 : Inport  Port=2
  In3 : Inport  Port=3
  In4 : Inport  Port=4
  In5 : Inport  Port=5
  In6 : Inport  Port=6
  In7 : Inport  Port=7
  In8 : Inport  Port=8
  In9 : Inport  Port=9
  In10 : Inport  Port=10
  In11 : Inport  Port=11
  In12 : Inport  Port=12
  Add{,4..7} (5 alike) : Sum  Inputs=+-
  Add3 : Sum
  Add8 : Sum
  Add9 : Sum
  Anode Pressure : Mux  Inputs=5
  Anode Temperature : Mux  Inputs=2
  Bus Creator3 : BusCreator  Inputs=12
  Cathode Pressure : Mux  Inputs=5
  Cathode Temperature : Mux  Inputs=6
  Constant5 : Constant  Value=273.15
  Constant6 : Constant  Value=1e5
  Coolant Pressure : Mux  Inputs=6
  From63 : From  Commented=on  GotoTag=CMP6520_P  TagVisibility=global
  From64 : From  Commented=on  GotoTag=CMP6520_rpm  TagVisibility=global
  From65 : From  Commented=on  GotoTag=Power_Stack  TagVisibility=global
  Gain : Gain  Gain=1e2
  Gain{1,3,5..10,12..14} (11 alike) : Gain  Gain=1e5
  Gain2 : Gain  Gain=1e2
  Gain4 : Gain  Gain=1e2
  Mux10 : Mux  Inputs=2
  Mux11 : Mux  Inputs=6
  Mux12 : Mux  Inputs=2
  Mux3 : Mux  Inputs=7
  Mux7 : Mux  Inputs=5
  Mux8 : Mux
  Mux9 : Mux  Inputs=3
  Out1 : Outport
  wires:
  [U_Stack_Cell_min] -> Mux7/1
  Gain9/1 -> Coolant Pressure/6
  [HT_outlet] -> Mux3/7
  [HT_inlet] -> Mux3/6
  [TT6812] -> Mux3/5
  [TT6820] -> Mux3/4
  [TT6801] -> Mux3/3
  Gain1/1 -> Coolant Pressure/5
  Gain12/1 -> Coolant Pressure/4
  Gain10/1 -> Coolant Pressure/3
  [PT6812] -> Gain1/1
  [TT6901] -> Cathode Temperature/6
  [TT6512] -> Cathode Temperature/5
  [TT6511] -> Cathode Temperature/4
  [EACi_temp] -> Cathode Temperature/3
  Gain14/1 -> Cathode Pressure/5
  Gain8/1 -> Cathode Pressure/4
  Gain7/1 -> Cathode Pressure/3
  Bus Creator3/1 -> Out1/1
  Mux11/1 -> Bus Creator3/12
  Mux12/1 -> Bus Creator3/11
  Mux8/1 -> Bus Creator3/8
  Mux7/1 -> Bus Creator3/7
  Mux3/1 -> Bus Creator3/6
  Coolant Pressure/1 -> Bus Creator3/5
  Cathode Temperature/1 -> Bus Creator3/4
  Cathode Pressure/1 -> Bus Creator3/3
  Anode Pressure/1 -> Bus Creator3/1
  [H2O_Transport] -> Mux11/3
  [S5_mdot_water_kgs_FCS_production] -> Mux11/2
  [S5_mdot_water_kgs_FCS_outlet] -> Mux11/1
  [S5_Hum_rel_FCS_outlet] -> Mux12/2
  [cathode_supply_relative_humidity] -> Mux12/1
  [Cathode_Stoichiometry] -> Mux10/2
  [Anode_Stoichiometry] -> Mux10/1
  [mdot_Stack_in_kgs] -> Mux9/3
  [anode_mdot_kgs] -> Mux9/2
  In12/1 -> Mux8/2
  In7/1 -> Mux7/5
  In5/1 -> Mux7/2
  In6/1 -> Mux7/4
  Add8/1 -> Mux3/2
  Add5/1 -> Cathode Temperature/2
  Add6/1 -> Coolant Pressure/2
  Add4/1 -> Cathode Pressure/2
  Gain6/1 -> Anode Pressure/4
  Add3/1 -> Anode Temperature/2
  Gain5/1 -> Anode Pressure/3
  Mux9/1 -> Bus Creator3/9
  Add/1 -> Anode Pressure/2
  Gain13/1 -> Anode Pressure/5
  In10/1 -> Add8/2
  In9/1 -> Mux7/3
  Add7/1 -> Mux3/1, Add8/1
  Gain4/1 -> Add6/2
  Add9/1 -> Coolant Pressure/1, Add6/1
  [PT6811] -> Gain12/1
  Mux10/1 -> Bus Creator3/10
  [PT6114] -> Gain13/1
  [PT6512] -> Gain14/1
  Anode Temperature/1 -> Bus Creator3/2
  In11/1 -> Mux8/1
  [PT6500] -> Gain7/1
  [PT6510] -> Gain8/1
  [PT6701] -> Gain9/1
  [PT6801] -> Gain10/1
  [PT6100] -> Gain5/1
  [PT6111] -> Gain6/1
  [Current_Stack] -> Mux8/3
  Gain3/1 -> Anode Pressure/1, Add/1
  Gain2/1 -> Add/2
  In8/1 -> Gain4/1
  Constant5/1 -> Add7/2
  Constant6/1 -> Add9/2
  [T_Stack_in_K] -> Add7/1
  [P_Stack_in_Pa] -> Add9/1
  In4/1 -> Add5/2
  [voltage_Stack] -> Mux8/4
  [Cathode_mdot_kgs] -> Mux9/1
  In3/1 -> Gain/1
  Gain/1 -> Add4/2
  In1/1 -> Gain2/1
  In2/1 -> Add3/2
  [cathode_inlet_pressure_Pa] -> Add4/1, Cathode Pressure/1
  [cathode_supply_temperature] -> Cathode Temperature/1, Add5/1
  [anode_inlet_pressure_bara] -> Gain3/1
  [anode_inlet_Temperature_degC] -> Anode Temperature/1, Add3/1

== matlab function stack_model_subsystem/Simulink Function/MATLAB Function ==
  data: moist_air_temperature input; relative_humidity input; dewpoint_temperature output
function dewpoint_temperature = approximate_dewpoint(moist_air_temperature, relative_humidity)
% This function approximates the dewpoint temperature of moist air
% according to the August–Roche–Magnus approximation of the
% Clausius–Clapeyron equation.
%
% Inputs: Relative Humidity [-], Moist Air Temperature [°C]
% Output: Dewpoint Temperature [°C]
%
% Reference: https://bmcnoldy.earth.miami.edu/Humidity.html, retrieved
% 09/07/2023

% clip to [0, 1] and convert to [%]
relative_humidity = min(max(0, relative_humidity), 1)*100;

% August–Roche–Magnus approximation
dewpoint_temperature = 243.04*(log(relative_humidity/100)+((17.625*moist_air_temperature)/(243.04+moist_air_temperature)))/...
    (17.625-log(relative_humidity/100)-((17.625*moist_air_temperature)/(243.04+moist_air_temperature)));
